simulink model "KUKA_EE_Controller_v22_orbital_verification2"  (R2024a)
settings: Solver=VariableStepAuto  StartTime=0.0  StopTime=120  FixedStep=0.01  RelTol=1e-3
InitFcn:
  | %rho_0t=[0.29;0.29;0.29]; %m
  | %V_0t=[-0.001;-0.001;0];%[-0.0005;-0.0005;0];
  | %w_t=[0;0;-0.002];
  | 
  | 
  | %rho_0t=[0.3;0.3;0.2]; %m
  | %V_0t=[-0.001;-0.001;0];%[-0.0005;-0.0005;0];
  | %w_t=[0;0;-0.001];
values from neighbouring files (symbols this model uses):
  e_orbit = 0    [Initiate_FQ.m]
  e_orbit_t = (mu_orbit_t^2/mu_earth)/radius_orbit_t-1    [Initiate_FQ.m]
  g_cm = zeros(4,4,n)    [Initiate_KUKA_inv.m]    (also in KUKA_Main.m)
  M0 = M_temp.M0.data(:,:,1)    [Initiate_FQ.m]    (also in KUKA_Main.m)
  m0 = robot.Bodies{1,n+1}.Mass    [Initiate_KUKA_inv.m]    (also in KUKA_Main.m)
  m0_frak = diag_M(1:6,1:6)    [Initiate_KUKA_inv.m]
  M0m = M_temp.M0m.data(:,:,1)    [Initiate_FQ.m]    (also in KUKA_Main.m)
  m_diag = diag_M(7:end,7:end)    [Initiate_KUKA_inv.m]
  Mean_Anomaly0 = MeanAnomaly(e_orbit,E0)    [Initiate_FQ.m]
  Mean_Anomaly0_t = MeanAnomaly(e_orbit,E0)    [Initiate_FQ.m]
  Mm = simplify(transpose(Xi_m)*transpose(Lm)*diagM*Lm*Xi_m)    [KUKA_Main.m]
  mm = zeros(1,n)    [Initiate_KUKA_inv.m]    (also in KUKA_Main.m)
  mu = P0    [Initiate_FQ.m]    (also in Initiate_KUKA_inv.m = zeros(6,1); KUKA_Main.m = P)
  mu_earth = 3.986004418*10^14    (= 398600441800000)    [Initiate_FQ.m]
  mu_orbit = sqrt(radius_orbit*mu_earth)    [Initiate_FQ.m]
  mu_orbit_t = radius_orbit_t*vel_orbit_t    [Initiate_FQ.m]
  n_orbit = (mu_earth^2)/(mu_orbit^3)    [Initiate_FQ.m]
  n_orbit_t = (mu_earth^2)/(mu_orbit^3)    [Initiate_FQ.m]
  q_dot_m = [0;0;0;0;0;0;0]    [Initiate_FQ.m]    (also in Initiate_KUKA_inv.m; KUKA_Main.m = [qdot1;qdot2;qdot3;qdot4;qdot5;qdot6;qdot7])
  q_m = [0.2;1.2;0.3;2.5;0.5;1.5;0.6]    [Initiate_FQ.m]    (also in Initiate_KUKA_inv.m = [0;0;0;0;0;0;0]; KUKA_Main.m = [q_m1;q_m2;q_m3;q_m4;q_m5;q_m6;q_m7])
  sc_size = 1    [Initiate_KUKA_inv.m]    (also in KUKA_Main.m)
  theta0 = 0    [Initiate_FQ.m]
  theta0_t = 0    [Initiate_FQ.m]
  V_I0 = [-0.0001;-0.0001;0.0;-0.001;0.001;0.002]    [Initiate_FQ.m]    (also in Initiate_KUKA_inv.m = [0;0;0;0;0;0]; KUKA_Main.m = [0;0;0;0;0;0])
  Xi_m = Xi_m(1:robot.n*6,1:robot.n)    [KUKA_Main.m]
  Xi_m_matrix = zeros(6*n,n)    [Initiate_KUKA_inv.m]    (also in KUKA_Main.m)
undefined symbols (not defined in the file or in its folder): g_cm0, I0, Im, X, Y, Z
libraries: nesl_utility x121, sm_lib x101, simulink x12, robotcorelib x7
(part 4 of 4)

== system KUKA_EE_Controller_v22_orbital_verification2/Space Manipulator1/joint//link7/iiwa_link_7 ==
  Inertia : sm_lib/Body Elements/Inertia  InertiaType=Custom  Mass=m0  MassUnits=kg  CenterOfMass=[0, 0, 0]  CenterOfMassUnits=m  MomentsOfInertia=[I0(1,1) I0(2,2) I0(3,3)]  MomentsOfInertiaUnits=kg*m^2  ProductsOfInertia=[I0(3,2) I0(3,1) I0(2,1)]  ProductsOfInertiaUnits=kg*m^2  GraphicType=None  MarkerShape=Inertia  MarkerSize=20  GraphicVisPropType=SimpleVisualProperties  GraphicDiffuseColor=[0.5 0.5 0.5]  GraphicOpacity=1.0  GraphicSpecularColor=[0.5 0.5 0.5 1.0]  GraphicAmbientColor=[0.15 0.15 0.15 1.0]  GraphicEmissiveColor=[0.0 0.0 0.0 1.0]  GraphicShininess=75
  Visual : sm_lib/Body Elements/File Solid  ExtGeomFileName=iiwa_description/meshes/iiwa7/visual/link_7.stl  UnitType=Custom  ExtGeomFileUnits=m  StepReaderType=HEX  ExportConvexHullGeometry=off  InertiaType=Custom  BasedOnType=DensityFromFile  Density=1000  DensityUnits=kg/m^3  Mass=0  MassUnits=kg  CenterOfMass=[0, 0, 0]  CenterOfMassUnits=m  MomentsOfInertia=[0, 0, 0]  MomentsOfInertiaUnits=kg*m^2  ProductsOfInertia=[0, 0, 0]  ProductsOfInertiaUnits=kg*m^2  GraphicType=FromGeometry  MarkerShape=Sphere  MarkerSize=10  GraphicVisPropType=SimpleVisualProperties  GraphicDiffuseColor=[0.4, 0.4, 0.4]  GraphicOpacity=1  GraphicSpecularColor=[0.5 0.5 0.5 1.0]  GraphicAmbientColor=[0.15 0.15 0.15 1.0]  GraphicEmissiveColor=[0.0 0.0 0.0 1.0]  GraphicShininess=75  DoExposeReferenceFrame=on  SerializedFrames=<Frames/>
  VisualOriginTransform : sm_lib/Frames and Transforms/Rigid Transform  RotationMethod=RotationSequence  FollAlignAxisA=+X  BaseAlignAxisA=+Y  FollAlignAxisB=+Y  BaseAlignAxisB=+Z  RotationStandardAxis=+Z  RotationAngle=0.0  RotationAngleUnits=deg  RotationArbitraryAxis=[0 0 1]  RotationSequenceAxes=BaseAxes  RotationSequence=XYZ  RotationSequenceAngles=[0, 0, 0]  RotationSequenceAnglesUnits=rad  RotationMatrix=[1 0 0; 0 1 0; 0 0 1]  Quaternion=[1 0 0 0]  TranslationMethod=Cartesian  TranslationCartesianOffset=[0, 0, 0]  TranslationCartesianOffsetUnits=m  TranslationStandardAxis=+Z  TranslationStandardOffset=0  TranslationStandardOffsetUnits=m  TranslationROffset=0  TranslationROffsetUnits=m  TranslationThetaOffset=0  TranslationThetaOffsetUnits=deg  TranslationZOffset=0  TranslationZOffsetUnits=m
  iiwa_joint_ee_OriginTransform : sm_lib/Frames and Transforms/Rigid Transform  RotationMethod=RotationMatrix  FollAlignAxisA=+X  BaseAlignAxisA=+Y  FollAlignAxisB=+Y  BaseAlignAxisB=+Z  RotationStandardAxis=+Z  RotationAngle=0.0  RotationAngleUnits=deg  RotationArbitraryAxis=[0 0 1]  RotationSequenceAxes=BaseAxes  RotationSequence=XYZ  RotationSequenceAngles=[0, 0, 0]  RotationSequenceAnglesUnits=rad  RotationMatrix=g_cm0(1:3,1:3)  Quaternion=[1 0 0 0]  TranslationMethod=Cartesian  TranslationCartesianOffset=g_cm0(1:3,4)'  TranslationCartesianOffsetUnits=m  TranslationStandardAxis=+Z  TranslationStandardOffset=0  TranslationStandardOffsetUnits=m  TranslationROffset=0  TranslationROffsetUnits=m  TranslationThetaOffset=0  TranslationThetaOffsetUnits=deg  TranslationZOffset=0  TranslationZOffsetUnits=m
  F : PMIOPort  Side=Left
  F1 : PMIOPort  Port=2  Side=Right
  connections:
  iiwa_joint_ee_OriginTransform/LConn1 -- F1/RConn1
  Visual/RConn1 -- VisualOriginTransform/RConn1
  Inertia/RConn1 -- VisualOriginTransform/LConn1 -- iiwa_joint_ee_OriginTransform/RConn1 -- F/RConn1

== system KUKA_EE_Controller_v22_orbital_verification2/Space Manipulator4/join//link 1/iiwa_link_1 ==
  Inertia : sm_lib/Body Elements/Inertia  InertiaType=Custom  Mass=mm(6)  MassUnits=kg  CenterOfMass=[0, 0, 0]  CenterOfMassUnits=m  MomentsOfInertia=[Im(1,1,6) Im(2,2,6) Im(3,3,6)]  MomentsOfInertiaUnits=kg*m^2  ProductsOfInertia=[Im(3,2,6) Im(3,1,6) Im(2,1,6)]  ProductsOfInertiaUnits=kg*m^2  GraphicType=None  MarkerShape=Inertia  MarkerSize=20  GraphicVisPropType=SimpleVisualProperties  GraphicDiffuseColor=[0.5 0.5 0.5]  GraphicOpacity=1.0  GraphicSpecularColor=[0.5 0.5 0.5 1.0]  GraphicAmbientColor=[0.15 0.15 0.15 1.0]  GraphicEmissiveColor=[0.0 0.0 0.0 1.0]  GraphicShininess=75
  Visual : sm_lib/Body Elements/File Solid  ExtGeomFileName=iiwa_description/meshes/iiwa7/visual/link_1.stl  UnitType=Custom  ExtGeomFileUnits=m  StepReaderType=HEX  ExportConvexHullGeometry=off  InertiaType=Custom  BasedOnType=DensityFromFile  Density=1000  DensityUnits=kg/m^3  Mass=0  MassUnits=kg  CenterOfMass=[0, 0, 0]  CenterOfMassUnits=m  MomentsOfInertia=[0, 0, 0]  MomentsOfInertiaUnits=kg*m^2  ProductsOfInertia=[0, 0, 0]  ProductsOfInertiaUnits=kg*m^2  GraphicType=FromGeometry  MarkerShape=Sphere  MarkerSize=10  GraphicVisPropType=SimpleVisualProperties  GraphicDiffuseColor=[1, 0.423529411765, 0.0392156862745]  GraphicOpacity=1  GraphicSpecularColor=[0.5 0.5 0.5 1.0]  GraphicAmbientColor=[0.15 0.15 0.15 1.0]  GraphicEmissiveColor=[0.0 0.0 0.0 1.0]  GraphicShininess=75  DoExposeReferenceFrame=on  SerializedFrames=<Frames/>
  VisualOriginTransform : sm_lib/Frames and Transforms/Rigid Transform  RotationMethod=RotationSequence  FollAlignAxisA=+X  BaseAlignAxisA=+Y  FollAlignAxisB=+Y  BaseAlignAxisB=+Z  RotationStandardAxis=+Z  RotationAngle=0.0  RotationAngleUnits=deg  RotationArbitraryAxis=[0 0 1]  RotationSequenceAxes=BaseAxes  RotationSequence=XYZ  RotationSequenceAngles=[0, 0, 0]  RotationSequenceAnglesUnits=rad  RotationMatrix=[1 0 0; 0 1 0; 0 0 1]  Quaternion=[1 0 0 0]  TranslationMethod=Cartesian  TranslationCartesianOffset=[0, 0, 0]  TranslationCartesianOffsetUnits=m  TranslationStandardAxis=+Z  TranslationStandardOffset=0  TranslationStandardOffsetUnits=m  TranslationROffset=0  TranslationROffsetUnits=m  TranslationThetaOffset=0  TranslationThetaOffsetUnits=deg  TranslationZOffset=0  TranslationZOffsetUnits=m
  iiwa_joint_2_OriginTransform : sm_lib/Frames and Transforms/Rigid Transform  RotationMethod=RotationMatrix  FollAlignAxisA=+X  BaseAlignAxisA=+Y  FollAlignAxisB=+Y  BaseAlignAxisB=+Z  RotationStandardAxis=+Z  RotationAngle=0.0  RotationAngleUnits=deg  RotationArbitraryAxis=[0 0 1]  RotationSequenceAxes=BaseAxes  RotationSequence=XYZ  RotationSequenceAngles=[1.57079632679, 0, 3.14159265359]  RotationSequenceAnglesUnits=rad  RotationMatrix=g_cm(1:3,1:3,6)  Quaternion=[1 0 0 0]  TranslationMethod=Cartesian  TranslationCartesianOffset=g_cm(1:3,4,6)'  TranslationCartesianOffsetUnits=m  TranslationStandardAxis=+Z  TranslationStandardOffset=0  TranslationStandardOffsetUnits=m  TranslationROffset=0  TranslationROffsetUnits=m  TranslationThetaOffset=0  TranslationThetaOffsetUnits=deg  TranslationZOffset=0  TranslationZOffsetUnits=m
  F : PMIOPort  Side=Left
  F1 : PMIOPort  Port=2  Side=Right
  connections:
  Visual/RConn1 -- VisualOriginTransform/RConn1
  VisualOriginTransform/LConn1 -- Inertia/RConn1 -- iiwa_joint_2_OriginTransform/RConn1 -- F/RConn1
  F1/RConn1 -- iiwa_joint_2_OriginTransform/LConn1

== system KUKA_EE_Controller_v22_orbital_verification2/Space Manipulator4/joint//link2/iiwa_link_2 ==
  Inertia : sm_lib/Body Elements/Inertia  InertiaType=Custom  Mass=mm(5)  MassUnits=kg  CenterOfMass=[0, 0, 0]  CenterOfMassUnits=m  MomentsOfInertia=[Im(1,1,5) Im(2,2,5) Im(3,3,5)]  MomentsOfInertiaUnits=kg*m^2  ProductsOfInertia=[Im(3,2,5) Im(3,1,5) Im(2,1,5)]  ProductsOfInertiaUnits=kg*m^2  GraphicType=None  MarkerShape=Inertia  MarkerSize=20  GraphicVisPropType=SimpleVisualProperties  GraphicDiffuseColor=[0.5 0.5 0.5]  GraphicOpacity=1.0  GraphicSpecularColor=[0.5 0.5 0.5 1.0]  GraphicAmbientColor=[0.15 0.15 0.15 1.0]  GraphicEmissiveColor=[0.0 0.0 0.0 1.0]  GraphicShininess=75
  Visual : sm_lib/Body Elements/File Solid  ExtGeomFileName=iiwa_description/meshes/iiwa7/visual/link_2.stl  UnitType=Custom  ExtGeomFileUnits=m  StepReaderType=HEX  ExportConvexHullGeometry=off  InertiaType=Custom  BasedOnType=DensityFromFile  Density=1000  DensityUnits=kg/m^3  Mass=0  MassUnits=kg  CenterOfMass=[0, 0, 0]  CenterOfMassUnits=m  MomentsOfInertia=[0, 0, 0]  MomentsOfInertiaUnits=kg*m^2  ProductsOfInertia=[0, 0, 0]  ProductsOfInertiaUnits=kg*m^2  GraphicType=FromGeometry  MarkerShape=Sphere  MarkerSize=10  GraphicVisPropType=SimpleVisualProperties  GraphicDiffuseColor=[1, 0.423529411765, 0.0392156862745]  GraphicOpacity=1  GraphicSpecularColor=[0.5 0.5 0.5 1.0]  GraphicAmbientColor=[0.15 0.15 0.15 1.0]  GraphicEmissiveColor=[0.0 0.0 0.0 1.0]  GraphicShininess=75  DoExposeReferenceFrame=on  SerializedFrames=<Frames/>
  VisualOriginTransform : sm_lib/Frames and Transforms/Rigid Transform  RotationMethod=RotationSequence  FollAlignAxisA=+X  BaseAlignAxisA=+Y  FollAlignAxisB=+Y  BaseAlignAxisB=+Z  RotationStandardAxis=+Z  RotationAngle=0.0  RotationAngleUnits=deg  RotationArbitraryAxis=[0 0 1]  RotationSequenceAxes=BaseAxes  RotationSequence=XYZ  RotationSequenceAngles=[0, 0, 0]  RotationSequenceAnglesUnits=rad  RotationMatrix=[1 0 0; 0 1 0; 0 0 1]  Quaternion=[1 0 0 0]  TranslationMethod=Cartesian  TranslationCartesianOffset=[0, 0, 0]  TranslationCartesianOffsetUnits=m  TranslationStandardAxis=+Z  TranslationStandardOffset=0  TranslationStandardOffsetUnits=m  TranslationROffset=0  TranslationROffsetUnits=m  TranslationThetaOffset=0  TranslationThetaOffsetUnits=deg  TranslationZOffset=0  TranslationZOffsetUnits=m
  iiwa_joint_3_OriginTransform : sm_lib/Frames and Transforms/Rigid Transform  RotationMethod=RotationMatrix  FollAlignAxisA=+X  BaseAlignAxisA=+Y  FollAlignAxisB=+Y  BaseAlignAxisB=+Z  RotationStandardAxis=+Z  RotationAngle=0.0  RotationAngleUnits=deg  RotationArbitraryAxis=[0 0 1]  RotationSequenceAxes=BaseAxes  RotationSequence=XYZ  RotationSequenceAngles=[1.57079632679, 0, 3.14159265359]  RotationSequenceAnglesUnits=rad  RotationMatrix=g_cm(1:3,1:3,5)  Quaternion=[1 0 0 0]  TranslationMethod=Cartesian  TranslationCartesianOffset=g_cm(1:3,4,5)'  TranslationCartesianOffsetUnits=m  TranslationStandardAxis=+Z  TranslationStandardOffset=0  TranslationStandardOffsetUnits=m  TranslationROffset=0  TranslationROffsetUnits=m  TranslationThetaOffset=0  TranslationThetaOffsetUnits=deg  TranslationZOffset=0  TranslationZOffsetUnits=m
  F : PMIOPort  Side=Left
  F1 : PMIOPort  Port=2  Side=Right
  connections:
  Visual/RConn1 -- VisualOriginTransform/RConn1
  VisualOriginTransform/LConn1 -- Inertia/RConn1 -- iiwa_joint_3_OriginTransform/RConn1 -- F/RConn1
  iiwa_joint_3_OriginTransform/LConn1 -- F1/RConn1

== system KUKA_EE_Controller_v22_orbital_verification2/Space Manipulator4/joint//link3/iiwa_link_3 ==
  Inertia : sm_lib/Body Elements/Inertia  InertiaType=Custom  Mass=mm(4)  MassUnits=kg  CenterOfMass=[0, 0, 0]  CenterOfMassUnits=m  MomentsOfInertia=[Im(1,1,4) Im(2,2,4) Im(3,3,4)]  MomentsOfInertiaUnits=kg*m^2  ProductsOfInertia=[Im(3,2,4) Im(3,1,4) Im(2,1,4)]  ProductsOfInertiaUnits=kg*m^2  GraphicType=None  MarkerShape=Inertia  MarkerSize=20  GraphicVisPropType=SimpleVisualProperties  GraphicDiffuseColor=[0.5 0.5 0.5]  GraphicOpacity=1.0  GraphicSpecularColor=[0.5 0.5 0.5 1.0]  GraphicAmbientColor=[0.15 0.15 0.15 1.0]  GraphicEmissiveColor=[0.0 0.0 0.0 1.0]  GraphicShininess=75
  Visual : sm_lib/Body Elements/File Solid  ExtGeomFileName=iiwa_description/meshes/iiwa7/visual/link_3.stl  UnitType=Custom  ExtGeomFileUnits=m  StepReaderType=HEX  ExportConvexHullGeometry=off  InertiaType=Custom  BasedOnType=DensityFromFile  Density=1000  DensityUnits=kg/m^3  Mass=0  MassUnits=kg  CenterOfMass=[0, 0, 0]  CenterOfMassUnits=m  MomentsOfInertia=[0, 0, 0]  MomentsOfInertiaUnits=kg*m^2  ProductsOfInertia=[0, 0, 0]  ProductsOfInertiaUnits=kg*m^2  GraphicType=FromGeometry  MarkerShape=Sphere  MarkerSize=10  GraphicVisPropType=SimpleVisualProperties  GraphicDiffuseColor=[1, 0.423529411765, 0.0392156862745]  GraphicOpacity=1  GraphicSpecularColor=[0.5 0.5 0.5 1.0]  GraphicAmbientColor=[0.15 0.15 0.15 1.0]  GraphicEmissiveColor=[0.0 0.0 0.0 1.0]  GraphicShininess=75  DoExposeReferenceFrame=on  SerializedFrames=<Frames/>
  VisualOriginTransform : sm_lib/Frames and Transforms/Rigid Transform  RotationMethod=RotationSequence  FollAlignAxisA=+X  BaseAlignAxisA=+Y  FollAlignAxisB=+Y  BaseAlignAxisB=+Z  RotationStandardAxis=+Z  RotationAngle=0.0  RotationAngleUnits=deg  RotationArbitraryAxis=[0 0 1]  RotationSequenceAxes=BaseAxes  RotationSequence=XYZ  RotationSequenceAngles=[0, 0, 0]  RotationSequenceAnglesUnits=rad  RotationMatrix=[1 0 0; 0 1 0; 0 0 1]  Quaternion=[1 0 0 0]  TranslationMethod=Cartesian  TranslationCartesianOffset=[0, 0, -0.026]  TranslationCartesianOffsetUnits=m  TranslationStandardAxis=+Z  TranslationStandardOffset=0  TranslationStandardOffsetUnits=m  TranslationROffset=0  TranslationROffsetUnits=m  TranslationThetaOffset=0  TranslationThetaOffsetUnits=deg  TranslationZOffset=0  TranslationZOffsetUnits=m
  iiwa_joint_4_OriginTransform : sm_lib/Frames and Transforms/Rigid Transform  RotationMethod=RotationMatrix  FollAlignAxisA=+X  BaseAlignAxisA=+Y  FollAlignAxisB=+Y  BaseAlignAxisB=+Z  RotationStandardAxis=+Z  RotationAngle=0.0  RotationAngleUnits=deg  RotationArbitraryAxis=[0 0 1]  RotationSequenceAxes=BaseAxes  RotationSequence=XYZ  RotationSequenceAngles=[1.57079632679, 0, 0]  RotationSequenceAnglesUnits=rad  RotationMatrix=g_cm(1:3,1:3,4)  Quaternion=[1 0 0 0]  TranslationMethod=Cartesian  TranslationCartesianOffset=g_cm(1:3,4,4)'  TranslationCartesianOffsetUnits=m  TranslationStandardAxis=+Z  TranslationStandardOffset=0  TranslationStandardOffsetUnits=m  TranslationROffset=0  TranslationROffsetUnits=m  TranslationThetaOffset=0  TranslationThetaOffsetUnits=deg  TranslationZOffset=0  TranslationZOffsetUnits=m
  F : PMIOPort  Side=Left
  F1 : PMIOPort  Port=2  Side=Right
  connections:
  VisualOriginTransform/LConn1 -- iiwa_joint_4_OriginTransform/RConn1 -- Inertia/RConn1 -- F/RConn1
  Visual/RConn1 -- VisualOriginTransform/RConn1
  iiwa_joint_4_OriginTransform/LConn1 -- F1/RConn1

== system KUKA_EE_Controller_v22_orbital_verification2/Space Manipulator4/joint//link4/iiwa_link_4 ==
  Inertia : sm_lib/Body Elements/Inertia  InertiaType=Custom  Mass=mm(3)  MassUnits=kg  CenterOfMass=[0, 0, 0]  CenterOfMassUnits=m  MomentsOfInertia=[Im(1,1,3) Im(2,2,3) Im(3,3,3)]  MomentsOfInertiaUnits=kg*m^2  ProductsOfInertia=[Im(3,2,3) Im(3,1,3) Im(2,1,3)]  ProductsOfInertiaUnits=kg*m^2  GraphicType=None  MarkerShape=Inertia  MarkerSize=20  GraphicVisPropType=SimpleVisualProperties  GraphicDiffuseColor=[0.5 0.5 0.5]  GraphicOpacity=1.0  GraphicSpecularColor=[0.5 0.5 0.5 1.0]  GraphicAmbientColor=[0.15 0.15 0.15 1.0]  GraphicEmissiveColor=[0.0 0.0 0.0 1.0]  GraphicShininess=75
  Visual : sm_lib/Body Elements/File Solid  ExtGeomFileName=iiwa_description/meshes/iiwa7/visual/link_4.stl  UnitType=Custom  ExtGeomFileUnits=m  StepReaderType=HEX  ExportConvexHullGeometry=off  InertiaType=Custom  BasedOnType=DensityFromFile  Density=1000  DensityUnits=kg/m^3  Mass=0  MassUnits=kg  CenterOfMass=[0, 0, 0]  CenterOfMassUnits=m  MomentsOfInertia=[0, 0, 0]  MomentsOfInertiaUnits=kg*m^2  ProductsOfInertia=[0, 0, 0]  ProductsOfInertiaUnits=kg*m^2  GraphicType=FromGeometry  MarkerShape=Sphere  MarkerSize=10  GraphicVisPropType=SimpleVisualProperties  GraphicDiffuseColor=[1, 0.423529411765, 0.0392156862745]  GraphicOpacity=1  GraphicSpecularColor=[0.5 0.5 0.5 1.0]  GraphicAmbientColor=[0.15 0.15 0.15 1.0]  GraphicEmissiveColor=[0.0 0.0 0.0 1.0]  GraphicShininess=75  DoExposeReferenceFrame=on  SerializedFrames=<Frames/>
  VisualOriginTransform : sm_lib/Frames and Transforms/Rigid Transform  RotationMethod=RotationSequence  FollAlignAxisA=+X  BaseAlignAxisA=+Y  FollAlignAxisB=+Y  BaseAlignAxisB=+Z  RotationStandardAxis=+Z  RotationAngle=0.0  RotationAngleUnits=deg  RotationArbitraryAxis=[0 0 1]  RotationSequenceAxes=BaseAxes  RotationSequence=XYZ  RotationSequenceAngles=[0, 0, 0]  RotationSequenceAnglesUnits=rad  RotationMatrix=[1 0 0; 0 1 0; 0 0 1]  Quaternion=[1 0 0 0]  TranslationMethod=Cartesian  TranslationCartesianOffset=[0, 0, 0]  TranslationCartesianOffsetUnits=m  TranslationStandardAxis=+Z  TranslationStandardOffset=0  TranslationStandardOffsetUnits=m  TranslationROffset=0  TranslationROffsetUnits=m  TranslationThetaOffset=0  TranslationThetaOffsetUnits=deg  TranslationZOffset=0  TranslationZOffsetUnits=m
  iiwa_joint_5_OriginTransform : sm_lib/Frames and Transforms/Rigid Transform  RotationMethod=RotationMatrix  FollAlignAxisA=+X  BaseAlignAxisA=+Y  FollAlignAxisB=+Y  BaseAlignAxisB=+Z  RotationStandardAxis=+Z  RotationAngle=0.0  RotationAngleUnits=deg  RotationArbitraryAxis=[0 0 1]  RotationSequenceAxes=BaseAxes  RotationSequence=XYZ  RotationSequenceAngles=[-1.57079632679, 3.14159265359, 0]  RotationSequenceAnglesUnits=rad  RotationMatrix=g_cm(1:3,1:3,3)  Quaternion=[1 0 0 0]  TranslationMethod=Cartesian  TranslationCartesianOffset=g_cm(1:3,4,3)'  TranslationCartesianOffsetUnits=m  TranslationStandardAxis=+Z  TranslationStandardOffset=0  TranslationStandardOffsetUnits=m  TranslationROffset=0  TranslationROffsetUnits=m  TranslationThetaOffset=0  TranslationThetaOffsetUnits=deg  TranslationZOffset=0  TranslationZOffsetUnits=m
  F : PMIOPort  Side=Left
  F1 : PMIOPort  Port=2  Side=Right
  connections:
  Visual/RConn1 -- VisualOriginTransform/RConn1
  VisualOriginTransform/LConn1 -- Inertia/RConn1 -- iiwa_joint_5_OriginTransform/RConn1 -- F/RConn1
  iiwa_joint_5_OriginTransform/LConn1 -- F1/RConn1

== system KUKA_EE_Controller_v22_orbital_verification2/Space Manipulator4/joint//link5/iiwa_link_5 ==
  Inertia : sm_lib/Body Elements/Inertia  InertiaType=Custom  Mass=mm(2)  MassUnits=kg  CenterOfMass=[0, 0, 0]  CenterOfMassUnits=m  MomentsOfInertia=[Im(1,1,2) Im(2,2,2) Im(3,3,2)]  MomentsOfInertiaUnits=kg*m^2  ProductsOfInertia=[Im(3,2,2) Im(3,1,2) Im(2,1,2)]  ProductsOfInertiaUnits=kg*m^2  GraphicType=None  MarkerShape=Inertia  MarkerSize=20  GraphicVisPropType=SimpleVisualProperties  GraphicDiffuseColor=[0.5 0.5 0.5]  GraphicOpacity=1.0  GraphicSpecularColor=[0.5 0.5 0.5 1.0]  GraphicAmbientColor=[0.15 0.15 0.15 1.0]  GraphicEmissiveColor=[0.0 0.0 0.0 1.0]  GraphicShininess=75
  Visual : sm_lib/Body Elements/File Solid  ExtGeomFileName=iiwa_description/meshes/iiwa7/visual/link_5.stl  UnitType=Custom  ExtGeomFileUnits=m  StepReaderType=HEX  ExportConvexHullGeometry=off  InertiaType=Custom  BasedOnType=DensityFromFile  Density=1000  DensityUnits=kg/m^3  Mass=0  MassUnits=kg  CenterOfMass=[0, 0, 0]  CenterOfMassUnits=m  MomentsOfInertia=[0, 0, 0]  MomentsOfInertiaUnits=kg*m^2  ProductsOfInertia=[0, 0, 0]  ProductsOfInertiaUnits=kg*m^2  GraphicType=FromGeometry  MarkerShape=Sphere  MarkerSize=10  GraphicVisPropType=SimpleVisualProperties  GraphicDiffuseColor=[1, 0.423529411765, 0.0392156862745]  GraphicOpacity=1  GraphicSpecularColor=[0.5 0.5 0.5 1.0]  GraphicAmbientColor=[0.15 0.15 0.15 1.0]  GraphicEmissiveColor=[0.0 0.0 0.0 1.0]  GraphicShininess=75  DoExposeReferenceFrame=on  SerializedFrames=<Frames/>
  VisualOriginTransform : sm_lib/Frames and Transforms/Rigid Transform  RotationMethod=RotationSequence  FollAlignAxisA=+X  BaseAlignAxisA=+Y  FollAlignAxisB=+Y  BaseAlignAxisB=+Z  RotationStandardAxis=+Z  RotationAngle=0.0  RotationAngleUnits=deg  RotationArbitraryAxis=[0 0 1]  RotationSequenceAxes=BaseAxes  RotationSequence=XYZ  RotationSequenceAngles=[0, 0, 0]  RotationSequenceAnglesUnits=rad  RotationMatrix=[1 0 0; 0 1 0; 0 0 1]  Quaternion=[1 0 0 0]  TranslationMethod=Cartesian  TranslationCartesianOffset=[0, 0, -0.026]  TranslationCartesianOffsetUnits=m  TranslationStandardAxis=+Z  TranslationStandardOffset=0  TranslationStandardOffsetUnits=m  TranslationROffset=0  TranslationROffsetUnits=m  TranslationThetaOffset=0  TranslationThetaOffsetUnits=deg  TranslationZOffset=0  TranslationZOffsetUnits=m
  iiwa_joint_6_OriginTransform : sm_lib/Frames and Transforms/Rigid Transform  Commented=on  RotationMethod=RotationSequence  FollAlignAxisA=+X  BaseAlignAxisA=+Y  FollAlignAxisB=+Y  BaseAlignAxisB=+Z  RotationStandardAxis=+Z  RotationAngle=0.0  RotationAngleUnits=deg  RotationArbitraryAxis=[0 0 1]  RotationSequenceAxes=BaseAxes  RotationSequence=XYZ  RotationSequenceAngles=[1.57079632679, 0, 0]  RotationSequenceAnglesUnits=rad  RotationMatrix=[1 0 0; 0 1 0; 0 0 1]  Quaternion=[1 0 0 0]  TranslationMethod=Cartesian  TranslationCartesianOffset=[0, 0.0607 , 0.19]  TranslationCartesianOffsetUnits=m  TranslationStandardAxis=+Z  TranslationStandardOffset=0  TranslationStandardOffsetUnits=m  TranslationROffset=0  TranslationROffsetUnits=m  TranslationThetaOffset=0  TranslationThetaOffsetUnits=deg  TranslationZOffset=0  TranslationZOffsetUnits=m
  iiwa_joint_6_OriginTransform1 : sm_lib/Frames and Transforms/Rigid Transform  RotationMethod=RotationMatrix  FollAlignAxisA=+X  BaseAlignAxisA=+Y  FollAlignAxisB=+Y  BaseAlignAxisB=+Z  RotationStandardAxis=+Z  RotationAngle=0.0  RotationAngleUnits=deg  RotationArbitraryAxis=[0 0 1]  RotationSequenceAxes=BaseAxes  RotationSequence=XYZ  RotationSequenceAngles=[1.57079632679, 0, 0]  RotationSequenceAnglesUnits=rad  RotationMatrix=g_cm(1:3,1:3,2)  Quaternion=[1 0 0 0]  TranslationMethod=Cartesian  TranslationCartesianOffset=g_cm(1:3,4,2)'  TranslationCartesianOffsetUnits=m  TranslationStandardAxis=+Z  TranslationStandardOffset=0  TranslationStandardOffsetUnits=m  TranslationROffset=0  TranslationROffsetUnits=m  TranslationThetaOffset=0  TranslationThetaOffsetUnits=deg  TranslationZOffset=0  TranslationZOffsetUnits=m
  F : PMIOPort  Side=Left
  F1 : PMIOPort  Port=2  Side=Right
  connections:
  Visual/RConn1 -- VisualOriginTransform/RConn1
  iiwa_joint_6_OriginTransform1/RConn1 -- Inertia/RConn1 -- VisualOriginTransform/LConn1 -- F/RConn1
  iiwa_joint_6_OriginTransform1/LConn1 -- F1/RConn1

== system KUKA_EE_Controller_v22_orbital_verification2/Space Manipulator4/joint//link6/iiwa_link_6 ==
  Inertia : sm_lib/Body Elements/Inertia  InertiaType=Custom  Mass=mm(1)  MassUnits=kg  CenterOfMass=[0, 0, 0]  CenterOfMassUnits=m  MomentsOfInertia=[Im(1,1,1) Im(2,2,1) Im(3,3,1)]  MomentsOfInertiaUnits=kg*m^2  ProductsOfInertia=[Im(3,2,1) Im(3,1,1) Im(2,1,1)]  ProductsOfInertiaUnits=kg*m^2  GraphicType=None  MarkerShape=Inertia  MarkerSize=20  GraphicVisPropType=SimpleVisualProperties  GraphicDiffuseColor=[0.5 0.5 0.5]  GraphicOpacity=1.0  GraphicSpecularColor=[0.5 0.5 0.5 1.0]  GraphicAmbientColor=[0.15 0.15 0.15 1.0]  GraphicEmissiveColor=[0.0 0.0 0.0 1.0]  GraphicShininess=75
  Visual : sm_lib/Body Elements/File Solid  ExtGeomFileName=iiwa_description/meshes/iiwa7/visual/link_6.stl  UnitType=Custom  ExtGeomFileUnits=m  StepReaderType=HEX  ExportConvexHullGeometry=off  InertiaType=Custom  BasedOnType=DensityFromFile  Density=1000  DensityUnits=kg/m^3  Mass=0  MassUnits=kg  CenterOfMass=[0, 0, 0]  CenterOfMassUnits=m  MomentsOfInertia=[0, 0, 0]  MomentsOfInertiaUnits=kg*m^2  ProductsOfInertia=[0, 0, 0]  ProductsOfInertiaUnits=kg*m^2  GraphicType=FromGeometry  MarkerShape=Sphere  MarkerSize=10  GraphicVisPropType=SimpleVisualProperties  GraphicDiffuseColor=[1, 0.423529411765, 0.0392156862745]  GraphicOpacity=1  GraphicSpecularColor=[0.5 0.5 0.5 1.0]  GraphicAmbientColor=[0.15 0.15 0.15 1.0]  GraphicEmissiveColor=[0.0 0.0 0.0 1.0]  GraphicShininess=75  DoExposeReferenceFrame=on  SerializedFrames=<Frames/>
  VisualOriginTransform : sm_lib/Frames and Transforms/Rigid Transform  RotationMethod=RotationSequence  FollAlignAxisA=+X  BaseAlignAxisA=+Y  FollAlignAxisB=+Y  BaseAlignAxisB=+Z  RotationStandardAxis=+Z  RotationAngle=0.0  RotationAngleUnits=deg  RotationArbitraryAxis=[0 0 1]  RotationSequenceAxes=BaseAxes  RotationSequence=XYZ  RotationSequenceAngles=[0, 0, 0]  RotationSequenceAnglesUnits=rad  RotationMatrix=[1 0 0; 0 1 0; 0 0 1]  Quaternion=[1 0 0 0]  TranslationMethod=Cartesian  TranslationCartesianOffset=[0, 0, 0.0607 ]  TranslationCartesianOffsetUnits=m  TranslationStandardAxis=+Z  TranslationStandardOffset=0  TranslationStandardOffsetUnits=m  TranslationROffset=0  TranslationROffsetUnits=m  TranslationThetaOffset=0  TranslationThetaOffsetUnits=deg  TranslationZOffset=0  TranslationZOffsetUnits=m
  iiwa_joint_7_OriginTransform : sm_lib/Frames and Transforms/Rigid Transform  RotationMethod=RotationMatrix  FollAlignAxisA=+X  BaseAlignAxisA=+Y  FollAlignAxisB=+Y  BaseAlignAxisB=+Z  RotationStandardAxis=+Z  RotationAngle=0.0  RotationAngleUnits=deg  RotationArbitraryAxis=[0 0 1]  RotationSequenceAxes=BaseAxes  RotationSequence=XYZ  RotationSequenceAngles=[-1.57079632679, 3.14159265359, 0]  RotationSequenceAnglesUnits=rad  RotationMatrix=g_cm(1:3,1:3,1)  Quaternion=[1 0 0 0]  TranslationMethod=Cartesian  TranslationCartesianOffset=g_cm(1:3,4,1)'  TranslationCartesianOffsetUnits=m  TranslationStandardAxis=+Z  TranslationStandardOffset=0  TranslationStandardOffsetUnits=m  TranslationROffset=0  TranslationROffsetUnits=m  TranslationThetaOffset=0  TranslationThetaOffsetUnits=deg  TranslationZOffset=0  TranslationZOffsetUnits=m
  F : PMIOPort  Side=Left
  F1 : PMIOPort  Port=2  Side=Right
  connections:
  iiwa_joint_7_OriginTransform/RConn1 -- Inertia/RConn1 -- F/RConn1 -- VisualOriginTransform/LConn1
  Visual/RConn1 -- VisualOriginTransform/RConn1
  iiwa_joint_7_OriginTransform/LConn1 -- F1/RConn1

== system KUKA_EE_Controller_v22_orbital_verification2/Space Manipulator4/joint//link7/iiwa_link_7 ==
  Inertia : sm_lib/Body Elements/Inertia  InertiaType=Custom  Mass=m0  MassUnits=kg  CenterOfMass=[0, 0, 0]  CenterOfMassUnits=m  MomentsOfInertia=[I0(1,1) I0(2,2) I0(3,3)]  MomentsOfInertiaUnits=kg*m^2  ProductsOfInertia=[I0(3,2) I0(3,1) I0(2,1)]  ProductsOfInertiaUnits=kg*m^2  GraphicType=None  MarkerShape=Inertia  MarkerSize=20  GraphicVisPropType=SimpleVisualProperties  GraphicDiffuseColor=[0.5 0.5 0.5]  GraphicOpacity=1.0  GraphicSpecularColor=[0.5 0.5 0.5 1.0]  GraphicAmbientColor=[0.15 0.15 0.15 1.0]  GraphicEmissiveColor=[0.0 0.0 0.0 1.0]  GraphicShininess=75
  Visual : sm_lib/Body Elements/File Solid  ExtGeomFileName=iiwa_description/meshes/iiwa7/visual/link_7.stl  UnitType=Custom  ExtGeomFileUnits=m  StepReaderType=HEX  ExportConvexHullGeometry=off  InertiaType=Custom  BasedOnType=DensityFromFile  Density=1000  DensityUnits=kg/m^3  Mass=0  MassUnits=kg  CenterOfMass=[0, 0, 0]  CenterOfMassUnits=m  MomentsOfInertia=[0, 0, 0]  MomentsOfInertiaUnits=kg*m^2  ProductsOfInertia=[0, 0, 0]  ProductsOfInertiaUnits=kg*m^2  GraphicType=FromGeometry  MarkerShape=Sphere  MarkerSize=10  GraphicVisPropType=SimpleVisualProperties  GraphicDiffuseColor=[0.4, 0.4, 0.4]  GraphicOpacity=1  GraphicSpecularColor=[0.5 0.5 0.5 1.0]  GraphicAmbientColor=[0.15 0.15 0.15 1.0]  GraphicEmissiveColor=[0.0 0.0 0.0 1.0]  GraphicShininess=75  DoExposeReferenceFrame=on  SerializedFrames=<Frames/>
  VisualOriginTransform : sm_lib/Frames and Transforms/Rigid Transform  RotationMethod=RotationSequence  FollAlignAxisA=+X  BaseAlignAxisA=+Y  FollAlignAxisB=+Y  BaseAlignAxisB=+Z  RotationStandardAxis=+Z  RotationAngle=0.0  RotationAngleUnits=deg  RotationArbitraryAxis=[0 0 1]  RotationSequenceAxes=BaseAxes  RotationSequence=XYZ  RotationSequenceAngles=[0, 0, 0]  RotationSequenceAnglesUnits=rad  RotationMatrix=[1 0 0; 0 1 0; 0 0 1]  Quaternion=[1 0 0 0]  TranslationMethod=Cartesian  TranslationCartesianOffset=[0, 0, 0]  TranslationCartesianOffsetUnits=m  TranslationStandardAxis=+Z  TranslationStandardOffset=0  TranslationStandardOffsetUnits=m  TranslationROffset=0  TranslationROffsetUnits=m  TranslationThetaOffset=0  TranslationThetaOffsetUnits=deg  TranslationZOffset=0  TranslationZOffsetUnits=m
  iiwa_joint_ee_OriginTransform : sm_lib/Frames and Transforms/Rigid Transform  RotationMethod=RotationMatrix  FollAlignAxisA=+X  BaseAlignAxisA=+Y  FollAlignAxisB=+Y  BaseAlignAxisB=+Z  RotationStandardAxis=+Z  RotationAngle=0.0  RotationAngleUnits=deg  RotationArbitraryAxis=[0 0 1]  RotationSequenceAxes=BaseAxes  RotationSequence=XYZ  RotationSequenceAngles=[0, 0, 0]  RotationSequenceAnglesUnits=rad  RotationMatrix=g_cm0(1:3,1:3)  Quaternion=[1 0 0 0]  TranslationMethod=Cartesian  TranslationCartesianOffset=g_cm0(1:3,4)'  TranslationCartesianOffsetUnits=m  TranslationStandardAxis=+Z  TranslationStandardOffset=0  TranslationStandardOffsetUnits=m  TranslationROffset=0  TranslationROffsetUnits=m  TranslationThetaOffset=0  TranslationThetaOffsetUnits=deg  TranslationZOffset=0  TranslationZOffsetUnits=m
  F : PMIOPort  Side=Left
  F1 : PMIOPort  Port=2  Side=Right
  connections:
  F/RConn1 -- iiwa_joint_ee_OriginTransform/RConn1 -- VisualOriginTransform/LConn1 -- Inertia/RConn1
  Visual/RConn1 -- VisualOriginTransform/RConn1
  iiwa_joint_ee_OriginTransform/LConn1 -- F1/RConn1

== matlab function KUKA_EE_Controller_v22_orbital_verification2/Space Manipulator4/collect positions1 ==
  data: g_ni output; g_n2 input; g_n3 input; g_n4 input; g_n5 input; g_n0 input
function g_ni = collect_poses(g_n2,g_n3,g_n4,g_n5, g_n0)

g_ni=zeros(4,4,4);
% p_joints=zeros(3,5);
g_ni(1,:,:)=g_n2;
g_ni(2,:,:)=g_n3;
g_ni(3,:,:)=g_n4;
g_ni(4,:,:)=g_n5;

== matlab function KUKA_EE_Controller_v22_orbital_verification2/Dynamic Parameters/MATLAB Function1 ==
  data: g_I0 input; mu input; P output
function P=Momentum(g_I0,mu)
% find the momentum in current base frame
P=Adjoint(g_I0)'*mu;

== matlab function KUKA_EE_Controller_v22_orbital_verification2/Dynamic Parameters/ 1 ==
  data: q_m input; L0 output; Lm0 output; Lm output; Xi_m input
function [L0,Lm0,Lm] =L_calculator(q_m,Xi_m)
% Calculates the time-dependent L matrix
n=length(q_m);
L=zeros(6*(n+1),6*(n+1));
% Compute M_frak for ith body
% Calculate L matrix
for i=1:n+1
    for j=1:n+1
        if i>j
            Ad_temp=eye(6);
            for k=j:i-1
                Ad_temp=Adjoint(g_Matrix(-Xi_m(:,k),q_m(k)))*Ad_temp;
            end
            L(6*(i-1)+1:6*(i-1)+6,6*(j-1)+1:6*(j-1)+6)=Ad_temp;
        elseif i==j
            L(6*(i-1)+1:6*(i-1)+6,6*(j-1)+1:6*(j-1)+6)=eye(6);
        elseif i<j
            L(6*(i-1)+1:6*(i-1)+6,6*(j-1)+1:6*(j-1)+6)=zeros(6);
        end
    end
end

L0=L(1:6,1:6);
Lm0=L(7:end,1:6);
Lm=L(7:end,7:end);

end

== matlab function KUKA_EE_Controller_v22_orbital_verification2/Space Manipulator4/Orbit/Orbit Pose ==
  data: t input; mu_orbit input; mu_earth input; e_orbit input; n_orbit input; theta0 input; R_orbit output; Mean_Anomaly0 input; p_orbit output; V_orbit_I output; theta_z output
function [R_orbit,p_orbit,V_orbit_I,theta_z] = V_orbit(t,mu_orbit, mu_earth, e_orbit,n_orbit,theta0, Mean_Anomaly0)


% Find current theta
theta=find_theta(t,e_orbit,n_orbit,Mean_Anomaly0);

% Find quasi-inertial frame velocity in perifocal
V_inertia_curly=(mu_earth/mu_orbit)*[-sin(theta0); e_orbit+cos(theta0);    0];
V_inertia=V_inertia_curly;

% Find relative velocity of orbit to quasi-inertial in perifocal
V_orbit=(mu_earth/mu_orbit)*[-sin(theta); e_orbit+cos(theta);    ((mu_earth)/(mu_orbit)^2)*(1+e_orbit*cos(theta))^2];
V_orbit_I=V_orbit-V_inertia;

% Find relative position of orbit to quasi-inertial frame in perifocal
p_orbit=(mu_orbit^2/mu_earth)/(1+e_orbit*cos(theta))*[cos(theta);sin(theta);0]              -(mu_orbit^2/mu_earth)/(1+e_orbit*cos(theta0))*[cos(theta0);sin(theta0);0]          -V_inertia*t;
%p_orbit=m_tot.*p_orbit;

% Find relative orientation of orbit to quasi-inertial frame in perifocal
R_orbit=[cos(theta-theta0) sin(theta-theta0) 0; -sin(theta-theta0) cos(theta-theta0) 0; 0 0 1];


% Find relative theta of orbit to quasi-inerital frame
theta_z=theta-theta0;




%-------------------------------------------------------------------
%temp
%E=0.5*MA_inv( Mean_Anomaly0 + (P_orb^(3/2)/mu_earth*t ));
%theta=2*atan(   ((1-e)/(1+e)) *tan(E));
%theta0=0;

%p_orbit=(mu_orbit^2/mu_earth)*[1/(1+e*cos(theta))-(cos(theta-theta0))/(1+e*cos(theta0)); (sin(theta-theta0))/(1+e*cos(theta0));   0];
%p_orbit=(mu_orbit^2/mu_earth)*[1/(1+e*cos(theta))-(cos(theta-theta0))/(1+e*cos(theta0)); (sin(theta-theta0))/(1+e*cos(theta0));   0];
%w_z=(mu_earth)^2/(mu_orbit^3)*(1+e_orbit*cos(theta))^2;

== matlab function KUKA_EE_Controller_v22_orbital_verification2/Space Manipulator4/Orbit/Orbit Pose1 ==
  data: t input; mu_orbit input; mu_earth input; e_orbit input; n input; theta0 input; R_orbit output; Mean_Anomaly0 input; p_orbit output; theta_z output; w_z output; mu_orbit_t input; e_orbit_t input; n_t input; theta0_t input; Mean_Anomaly0_t input
function [R_orbit,p_orbit,theta_z,w_z] = V_orbit(t,mu_orbit, mu_earth, e_orbit,n,theta0, Mean_Anomaly0, mu_orbit_t, e_orbit_t,n_t,theta0_t, Mean_Anomaly0_t)

theta=find_theta(t,e_orbit,n,Mean_Anomaly0);

%E=0.5*MA_inv( Mean_Anomaly0 + (P_orb^(3/2)/mu_earth*t ));
%theta=2*atan(   ((1-e)/(1+e)) *tan(E));
%theta0=0;

%p_orbit=(mu_orbit^2/mu_earth)*[1/(1+e*cos(theta))-(cos(theta-theta0))/(1+e*cos(theta0)); (sin(theta-theta0))/(1+e*cos(theta0));   0];
V_inertia_curly=(mu_earth/mu_orbit)*[-sin(theta0); e_orbit+cos(theta0);    0];

V_inertia=V_inertia_curly;

%p_orbit=(mu_orbit^2/mu_earth)*[1/(1+e*cos(theta))-(cos(theta-theta0))/(1+e*cos(theta0)); (sin(theta-theta0))/(1+e*cos(theta0));   0];
p_orbit=(mu_orbit^2/mu_earth)/(1+e_orbit*cos(theta))*([cos(theta);sin(theta);0]-[cos(theta0);sin(theta0);0])-V_inertia*t;
R_orbit=[cos(theta-theta0) sin(theta-theta0) 0; -sin(theta-theta0) cos(theta-theta0) 0; 0 0 1];

theta_z=theta-theta0;
w_z=(mu_earth)^2/(mu_orbit^3)*(1+e_orbit*cos(theta))^2;

%-------------------------------------------

theta_t=find_theta(t,e_orbit_t,n_t,Mean_Anomaly0_t);

%E=0.5*MA_inv( Mean_Anomaly0 + (P_orb^(3/2)/mu_earth*t ));
%theta=2*atan(   ((1-e)/(1+e)) *tan(E));
%theta0=0;

%p_orbit=(mu_orbit^2/mu_earth)*[1/(1+e*cos(theta))-(cos(theta-theta0))/(1+e*cos(theta0)); (sin(theta-theta0))/(1+e*cos(theta0));   0];
V_inertia_curly_t=(mu_earth/mu_orbit_t)*[-sin(theta0_t); e_orbit_t+cos(theta0_t);    0];

V_inertia_t=V_inertia_curly_t;

%p_orbit=(mu_orbit^2/mu_earth)*[1/(1+e*cos(theta))-(cos(theta-theta0))/(1+e*cos(theta0)); (sin(theta-theta0))/(1+e*cos(theta0));   0];
p_orbit_t=(mu_orbit_t^2/mu_earth)/(1+e_orbit_t*cos(theta_t))*([cos(theta_t);sin(theta_t);0]-[cos(theta0_t);sin(theta0_t);0])-V_inertia_t*t;
R_orbit_t=[cos(theta_t-theta0_t) sin(theta_t-theta0_t) 0; -sin(theta_t-theta0_t) cos(theta_t-theta0_t) 0; 0 0 1];

theta_z_t=theta_t-theta0_t;
w_z_t=(mu_earth)^2/(mu_orbit_t^3)*(1+e_orbit_t*cos(theta_t))^2;

p_orbit=p_orbit-p_orbit_t;
theta_z=theta_z-theta_z_t;

== matlab function KUKA_EE_Controller_v22_orbital_verification2/Space Manipulator1/Orbit/Orbit Pose ==
  data: t input; mu_orbit input; mu_earth input; e_orbit input; n_orbit input; theta0 input; R_orbit output; Mean_Anomaly0 input; p_orbit output; V_orbit_I output; theta_z output
function [R_orbit,p_orbit,V_orbit_I,theta_z] = V_orbit(t,mu_orbit, mu_earth, e_orbit,n_orbit,theta0, Mean_Anomaly0)


% Find current theta
theta=find_theta(t,e_orbit,n_orbit,Mean_Anomaly0);

% Find quasi-inertial frame velocity in perifocal
V_inertia_curly=(mu_earth/mu_orbit)*[-sin(theta0); e_orbit+cos(theta0);    0];
V_inertia=V_inertia_curly;

% Find relative velocity of orbit to quasi-inertial in perifocal
V_orbit=(mu_earth/mu_orbit)*[-sin(theta); e_orbit+cos(theta);    ((mu_earth)/(mu_orbit)^2)*(1+e_orbit*cos(theta))^2];
V_orbit_I=V_orbit-V_inertia;

% Find relative position of orbit to quasi-inertial frame in perifocal
p_orbit=(mu_orbit^2/mu_earth)/(1+e_orbit*cos(theta))*[cos(theta);sin(theta);0]              -(mu_orbit^2/mu_earth)/(1+e_orbit*cos(theta0))*[cos(theta0);sin(theta0);0]          -V_inertia*t;
%p_orbit=m_tot.*p_orbit;

% Find relative orientation of orbit to quasi-inertial frame in perifocal
R_orbit=[cos(theta-theta0) sin(theta-theta0) 0; -sin(theta-theta0) cos(theta-theta0) 0; 0 0 1];


% Find relative theta of orbit to quasi-inerital frame
theta_z=theta-theta0;




%-------------------------------------------------------------------
%temp
%E=0.5*MA_inv( Mean_Anomaly0 + (P_orb^(3/2)/mu_earth*t ));
%theta=2*atan(   ((1-e)/(1+e)) *tan(E));
%theta0=0;

%p_orbit=(mu_orbit^2/mu_earth)*[1/(1+e*cos(theta))-(cos(theta-theta0))/(1+e*cos(theta0)); (sin(theta-theta0))/(1+e*cos(theta0));   0];
%p_orbit=(mu_orbit^2/mu_earth)*[1/(1+e*cos(theta))-(cos(theta-theta0))/(1+e*cos(theta0)); (sin(theta-theta0))/(1+e*cos(theta0));   0];
%w_z=(mu_earth)^2/(mu_orbit^3)*(1+e_orbit*cos(theta))^2;

== matlab function KUKA_EE_Controller_v22_orbital_verification2/Space Manipulator1/Orbit/Orbit Pose1 ==
  data: t input; mu_orbit input; mu_earth input; e_orbit input; n input; theta0 input; R_orbit output; Mean_Anomaly0 input; p_orbit output; theta_z output; w_z output; mu_orbit_t input; e_orbit_t input; n_t input; theta0_t input; Mean_Anomaly0_t input
function [R_orbit,p_orbit,theta_z,w_z] = V_orbit(t,mu_orbit, mu_earth, e_orbit,n,theta0, Mean_Anomaly0, mu_orbit_t, e_orbit_t,n_t,theta0_t, Mean_Anomaly0_t)

theta=find_theta(t,e_orbit,n,Mean_Anomaly0);

%E=0.5*MA_inv( Mean_Anomaly0 + (P_orb^(3/2)/mu_earth*t ));
%theta=2*atan(   ((1-e)/(1+e)) *tan(E));
%theta0=0;

%p_orbit=(mu_orbit^2/mu_earth)*[1/(1+e*cos(theta))-(cos(theta-theta0))/(1+e*cos(theta0)); (sin(theta-theta0))/(1+e*cos(theta0));   0];
V_inertia_curly=(mu_earth/mu_orbit)*[-sin(theta0); e_orbit+cos(theta0);    0];

V_inertia=V_inertia_curly;

%p_orbit=(mu_orbit^2/mu_earth)*[1/(1+e*cos(theta))-(cos(theta-theta0))/(1+e*cos(theta0)); (sin(theta-theta0))/(1+e*cos(theta0));   0];
p_orbit=(mu_orbit^2/mu_earth)/(1+e_orbit*cos(theta))*([cos(theta);sin(theta);0]-[cos(theta0);sin(theta0);0])-V_inertia*t;
R_orbit=[cos(theta-theta0) sin(theta-theta0) 0; -sin(theta-theta0) cos(theta-theta0) 0; 0 0 1];

theta_z=theta-theta0;
w_z=(mu_earth)^2/(mu_orbit^3)*(1+e_orbit*cos(theta))^2;

%-------------------------------------------

theta_t=find_theta(t,e_orbit_t,n_t,Mean_Anomaly0_t);

%E=0.5*MA_inv( Mean_Anomaly0 + (P_orb^(3/2)/mu_earth*t ));
%theta=2*atan(   ((1-e)/(1+e)) *tan(E));
%theta0=0;

%p_orbit=(mu_orbit^2/mu_earth)*[1/(1+e*cos(theta))-(cos(theta-theta0))/(1+e*cos(theta0)); (sin(theta-theta0))/(1+e*cos(theta0));   0];
V_inertia_curly_t=(mu_earth/mu_orbit_t)*[-sin(theta0_t); e_orbit_t+cos(theta0_t);    0];

V_inertia_t=V_inertia_curly_t;

%p_orbit=(mu_orbit^2/mu_earth)*[1/(1+e*cos(theta))-(cos(theta-theta0))/(1+e*cos(theta0)); (sin(theta-theta0))/(1+e*cos(theta0));   0];
p_orbit_t=(mu_orbit_t^2/mu_earth)/(1+e_orbit_t*cos(theta_t))*([cos(theta_t);sin(theta_t);0]-[cos(theta0_t);sin(theta0_t);0])-V_inertia_t*t;
R_orbit_t=[cos(theta_t-theta0_t) sin(theta_t-theta0_t) 0; -sin(theta_t-theta0_t) cos(theta_t-theta0_t) 0; 0 0 1];

theta_z_t=theta_t-theta0_t;
w_z_t=(mu_earth)^2/(mu_orbit_t^3)*(1+e_orbit_t*cos(theta_t))^2;

p_orbit=p_orbit-p_orbit_t;
theta_z=theta_z-theta_z_t;

== matlab function KUKA_EE_Controller_v22_orbital_verification2/Space Manipulator1/Orbit/Orbit Pose2 ==
  data: q_dot input; A input; A_partial input; g_orbit_0 input; P_orbit_orbit input; N_orbit output; P_dot_orbit_orbit input
function N_orbit =N_orbit(q_dot,A,A_partial,g_orbit_0,P_orbit_orbit,P_dot_orbit_orbit)
% Calculate the N_hat_Orbit for the coupling of orbit/space manipulator

P_orbit=transpose(Adjoint(g_orbit_0))*P_orbit_orbit;

% ------------------ term 1 in N_orbit
N1_orbit=A'*transpose(adjoint_low(V))*transpose(Adjoint(g_orbit_0))*P_orbit_orbit;

% ------------------ term 2 in N_orbit
N2_orbit=A'*transpose(Adjoint(g_orbit_0))*P_dot_orbit_orbit;

% ------------------ term 3 in N_orbit
N3_orbit=zeros(); %insert dimension
temp=zeros(); %insert dimension
for i=1:n %n is number of joints
    temp=temp+(A_partial(i).*q_dot(i));
end
N3_orbit=-temp'*P_orbit;

% ------------------ term 4 in N_orbit
temp2=zeros(); %insert dimension
for i=1:n
    temp2(i,:)=q_dot'*A_partial(i)';
end
N4_orbit=temp2*P_orbit;

%  ------------------ term 5 in N_orbit

N_orbit=N1_orbit+N2_orbit+N3_orbit+N4_orbit;

== matlab function KUKA_EE_Controller_v22_orbital_verification2/Dynamic Parameters/MATLAB Function ==
  data: A input; wt output
function wt = fcn(A)

J=-A;
% SVD=svd(J);

% minSVD=min(SVD);
% maxSVD=max(SVD);

wt=sqrt(det(J*J'));

% y = minSVD/maxSVD;

== matlab function KUKA_EE_Controller_v22_orbital_verification2/Dynamic Parameters/V_I1 ==
  data: P input; A_connection input; q_dot_m input; M0 input; V_I0 output; g_I0 input
function V_I0 = V_I0(P, A_connection, q_dot_m, M0, g_I0)
V_I0=Adjoint(g_I0)*((M0\P)-A_connection*q_dot_m);

== matlab function KUKA_EE_Controller_v22_orbital_verification2/Space Manipulator4/collect positions ==
  data: p_ni output; p_n2 input; p_n3 input; p_n4 input; p_n5 input; g_n0 input
function p_ni = collect_positions(p_n2,p_n3,p_n4,p_n5, g_n0)

% R_0n=g_n0(1:3,1:3);
% p_0n=g_n0(1:3,4);

% p_joints=zeros(3,5);
p_ni=[p_n2 p_n3 p_n4  p_n5];
% p_joints=p_joints_temp(1:3,:);
